simulink model "Inverted_Pendulum"  (R2021a)
settings: Solver=FixedStepAuto  StartTime=0.0  StopTime=10  FixedStep=0.01  RelTol=1e-3
settings Model: Creator=sidhantdas  LastModifiedBy=sidhantdas

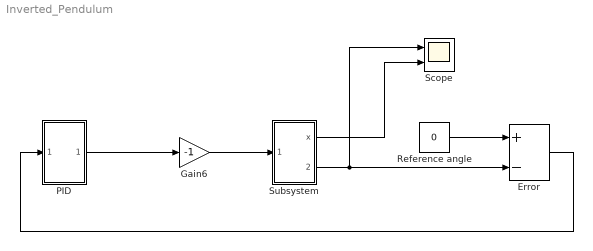
== system Inverted_Pendulum ==
  Error : Sum  Inputs=+-
  Gain6 : Gain  Gain=-1
  PID : Subsystem
  Reference angle : Constant  Value=0
  Scope : Scope  NumInputPorts=2
  Subsystem : Subsystem
  wires:
  Error/1 -> PID/1(In1)
  Gain6/1 -> Subsystem/1(Force)
  Reference angle/1 -> Error/1
  PID/1(Out1) -> Gain6/1
  Subsystem/2(theta) -> Scope/1, Error/2
  Subsystem/1(x) -> Scope/2

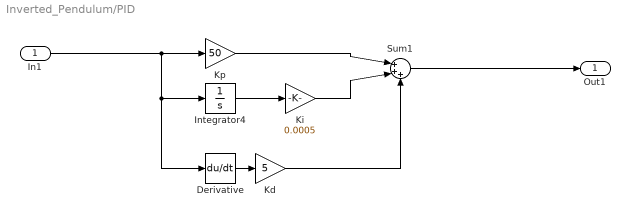
== system Inverted_Pendulum/PID ==
  In1 : Inport
  Derivative : Derivative
  Integrator4 : Integrator
  Kd : Gain  Gain=5
  Ki : Gain  Gain=0.0005
  Kp : Gain  Gain=50
  Sum1 : Sum  Inputs=|+++
  Out1 : Outport
  wires:
  Kp/1 -> Sum1/1
  Sum1/1 -> Out1/1
  Ki/1 -> Sum1/2
  In1/1 -> Derivative/1, Integrator4/1, Kp/1
  Derivative/1 -> Kd/1
  Kd/1 -> Sum1/3
  Integrator4/1 -> Ki/1

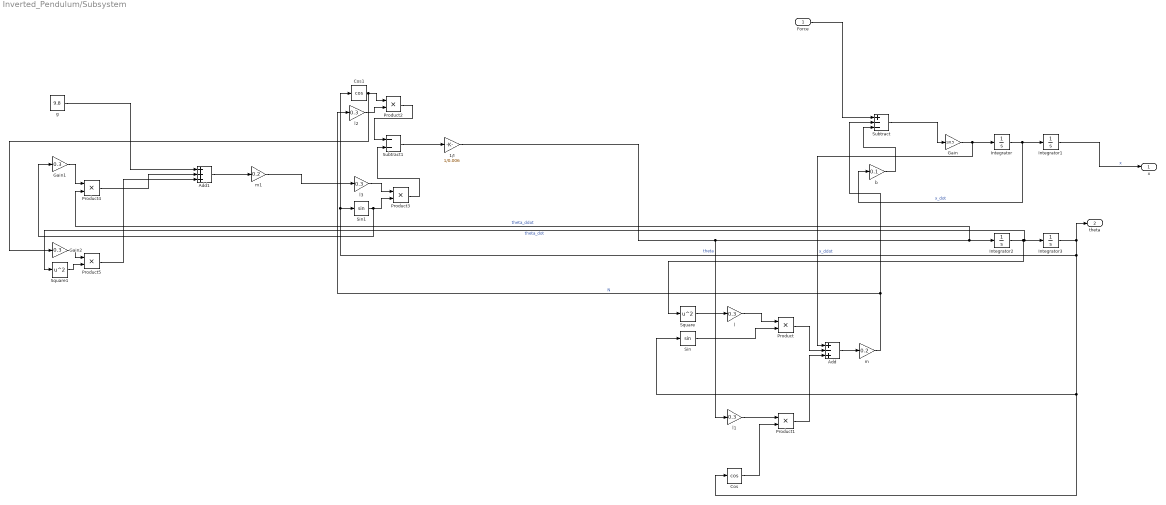
== system Inverted_Pendulum/Subsystem ==
  Force : Inport
  1/I : Gain  Gain=1/0.006
  Add : Sum  Inputs=+-+
  Add1 : Sum  Inputs=+++
  Cos : Trigonometry  Operator=cos
  Cos1 : Trigonometry  Operator=cos
  Gain : Gain  Gain=1/0.5
  Gain1 : Gain  Gain=0.3
  Gain2 : Gain  Gain=0.3
  Integrator : Integrator
  Integrator1 : Integrator
  Integrator2 : Integrator
  Integrator3 : Integrator  InitialCondition=0.17
  Product{,1..5} (6 alike) : Product
  Sin : Trigonometry
  Sin1 : Trigonometry
  Square : Math  Operator=square  SignedPower=on  SaturateOnIntegerOverflow=on
  Square1 : Math  Operator=square  SignedPower=on  SaturateOnIntegerOverflow=on
  Subtract : Sum  Inputs=+--
  Subtract1 : Sum  Inputs=--
  b : Gain  Gain=0.1
  g : Constant  Value=9.8
  l : Gain  Gain=0.3
  "l1 " : Gain  Gain=0.3
  l2 : Gain  Gain=0.3
  l3 : Gain  Gain=0.3
  "m " : Gain  Gain=0.2
  m1 : Gain  Gain=0.2
  x : Outport
  theta : Outport  Port=2
  wires:
  Integrator1/1 -> x/1  "x"
  Product4/1 -> Add1/2
  l3/1 -> Product3/1
  Subtract1/1 -> 1/I/1
  Subtract/1 -> Gain/1
  Square1/1 -> Product5/2
  Add/1 -> "m "/1
  Integrator3/1 -> theta/1, Cos1/1, Sin1/1, Cos/1, Sin/1  "theta"
  g/1 -> Add1/1
  Product1/1 -> Add/3
  Cos/1 -> Product1/2
  "l1 "/1 -> Product1/1
  Cos1/1 -> Gain2/1, Product2/1
  b/1 -> Subtract/3
  Product3/1 -> Subtract1/2
  Square/1 -> l/1
  l2/1 -> Product2/2
  Integrator/1 -> Integrator1/1, b/1  "x_dot"
  Product2/1 -> Subtract1/1
  Product5/1 -> Add1/3
  "m "/1 -> l2/1, Subtract/2  "N"
  Gain2/1 -> Product5/1
  m1/1 -> l3/1
  Integrator2/1 -> Square/1, Square1/1, Integrator3/1  "theta_dot"
  1/I/1 -> Product4/2, Integrator2/1, "l1 "/1  "theta_ddot"
  Product/1 -> Add/2
  Gain/1 -> Add/1, Integrator/1  "x_ddot"
  Sin1/1 -> Gain1/1, Product3/2
  Add1/1 -> m1/1
  l/1 -> Product/1
  Sin/1 -> Product/2
  Force/1 -> Subtract/1
  Gain1/1 -> Product4/1
